simulink model "Main_A"  (R2021a)
settings: Solver=daessc  StartTime=0.0  StopTime=20  RelTol=1e-3
model workspace (MAT data in the model file):
  VEH : object (value not decoded)
symbols that are objects in the model workspace (value not decoded): VEH
undefined symbols (not defined in the file): dT, Mu, MuSplit, P_ABSPressureRateMax, P_BrakePressureMax, P_PedalTravelRateMax, P_RefLine4SplitMue, P_RefLine_On, P_RefLineIsX, P_SplitMu_On, P_SplitMuOnlyAtBraking, P_SteeringMax, P_TorqueMax, t_Brake
libraries: sim3dlib x2, simulink_extras x1, vehdynlibsteering x1, sim3dautolib x1, simulink x1, vehdynlibviscommon x1
(part 2 of 2)

== matlab function Main_A/BrakeController/ECU ==
  data: Enable input; dT input; pMC input; WSS input; IMU input; pWhl output; MEM input; MEM_out output; Vel output; Desl output; YawRate output; LatAcc output; Yaw output; control output; tiempo output; Velmax output; ddd output
function [pWhl, MEM_out,Vel,Desl,YawRate,LatAcc,Yaw,control,tiempo,Velmax,ddd]= fcn(Enable, dT, pMC, WSS, IMU, MEM)

% ****************************** IMPORTANT ****************************** %
% NO work has to be done here. NO need to change this script, unless you
% need a different interface (i.e. inputs/outputs) to design or debug your
% controller.
% This function block only serves as a bridge to ABSfcn.m, so the
% controller's script (ABSfcn.m) can be stored in a file independent from
% the simulink model.
% *********************************************************************** %

% ******************************* INPUTS: ******************************* %
% Enable --> Switch to enable/disable controller (logic bit)              %
% Refer to ABSfcn.m for details regarding the rest of inputs              %
% *********************************************************************** %

% ************************ CASE: PASSIVE BRAKING ************************ %
% Passive braking means no control, whatsoever. Master cylinder pressure  %
% is equally passed to all wheels, same brake pressure across the         %
% multiple brake lines.                                                   %
if not(Enable)
    [pWhl, MEM_out,Vel,Desl,YawRate,LatAcc,Yaw,control,tiempo,Velmax,ddd] = ABSfcn(dT, pMC, WSS, IMU, MEM);
    
    
    
    pWhl    = [pMC pMC pMC pMC]';
    %MEM_out = zeros(50,1);
    
    return; % Exit function and do not run the rest of lines
end
% ********************* CASE: PASSIVE BRAKING - END ********************* %


% ********************** CASE: ABS CONTROL ENABLED ********************** %
[pWhl, MEM_out,Vel,Desl,YawRate,LatAcc,Yaw,control,tiempo,Velmax,ddd] = ABSfcn(dT, pMC, WSS, IMU, MEM);
% ******************* CASE: ABS CONTROL ENABLED - END ******************* %

end
